simulink model "lab6"  (R2019a)
settings: Solver=VariableStepAuto  StartTime=0.0  StopTime=10.0  RelTol=1e-3
settings Model: Creator=sumli  LastModifiedBy=sumli

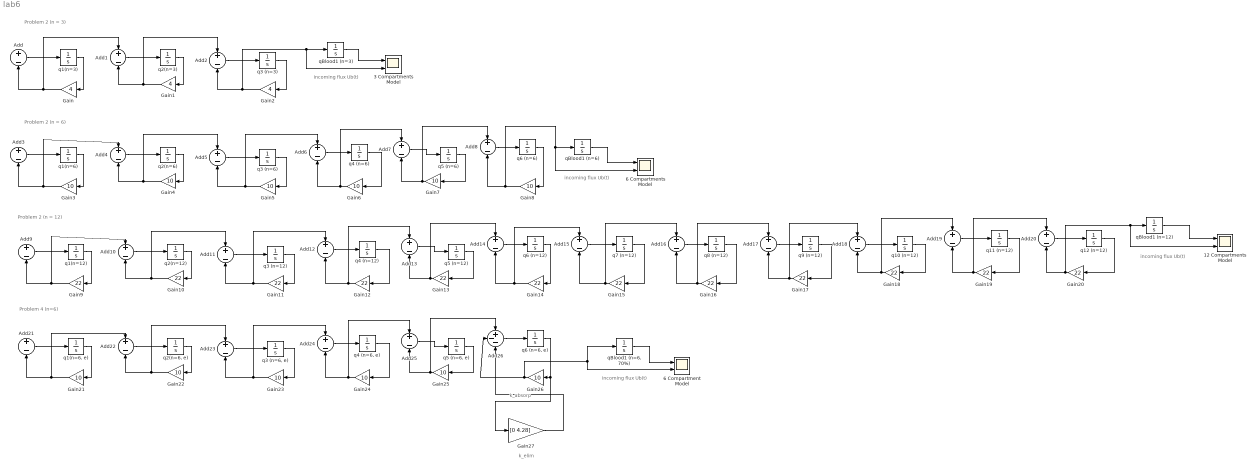
== system lab6 ==
  note: k_elim
  note: k_absorp
  note: incoming flux Ub(t)
  note: Problem 4 (n=6)
  note: Problem 2 (n = 12)
  note: Problem 2 (n = 6)
  note: Problem 2 (n = 3)
  note: incoming flux Ub(t)
  note: incoming flux Ub(t)
  note: incoming flux Ub(t)
  12 Compartments Model : Scope  NumInputPorts=2
  3 Compartments Model : Scope  NumInputPorts=2
  "6 Compartment Model " : Scope  NumInputPorts=2
  6 Compartments Model : Scope  NumInputPorts=2
  Add{,1..25} (26 alike) : Sum  Inputs=+-
  Add26 : Sum  Inputs=+--
  Gain : Gain  Gain=4
  Gain1 : Gain  Gain=4
  Gain{9..20} (12 alike) : Gain  Gain=22
  Gain2 : Gain  Gain=4
  Gain{3..8,21..26} (12 alike) : Gain  Gain=10
  Gain27 : Gain  Gain=[0 4.28]
  q1(n=12) : Integrator  InitialCondition=2
  q1(n=3) : Integrator  InitialCondition=2
  q1(n=6) : Integrator  InitialCondition=2
  "q1(n=6, e)" : Integrator  InitialCondition=2
  q10 (n=12) : Integrator
  q11 (n=12) : Integrator
  q12 (n=12) : Integrator
  q2(n=12) : Integrator
  q2(n=3) : Integrator
  q2(n=6) : Integrator
  "q2(n=6, e)" : Integrator
  q3 (n=12) : Integrator
  q3 (n=3) : Integrator
  q3 (n=6) : Integrator
  "q3 (n=6, e)" : Integrator
  q4 (n=12) : Integrator
  q4 (n=6) : Integrator
  "q4 (n=6, e)" : Integrator
  q5 (n=12) : Integrator
  q5 (n=6) : Integrator
  "q5 (n=6, e)" : Integrator
  q6 (n=12) : Integrator
  q6 (n=6) : Integrator
  "q6 (n=6, e)" : Integrator
  q7 (n=12) : Integrator
  q8 (n=12) : Integrator
  q9 (n=12) : Integrator
  qBlood1 (n=12) : Integrator
  qBlood1 (n=3) : Integrator
  qBlood1 (n=6) : Integrator
  "qBlood1 (n=6, 70%) " : Integrator
  wires:
  Add/1 -> q1(n=3)/1
  q1(n=3)/1 -> Gain/1
  Gain/1 -> Add1/1, Add/2
  Add1/1 -> q2(n=3)/1
  q2(n=3)/1 -> Gain1/1
  Gain1/1 -> Add2/1, Add1/2
  q3 (n=3)/1 -> Gain2/1
  Add2/1 -> q3 (n=3)/1
  Gain2/1 -> 3 Compartments Model/2, qBlood1 (n=3)/1, Add2/2
  qBlood1 (n=3)/1 -> 3 Compartments Model/1
  Gain3/1 -> Add4/1, Add3/2
  Add3/1 -> q1(n=6)/1
  Add5/1 -> q3 (n=6)/1
  Add4/1 -> q2(n=6)/1
  q3 (n=6)/1 -> Gain5/1
  q1(n=6)/1 -> Gain3/1
  q2(n=6)/1 -> Gain4/1
  Gain4/1 -> Add5/1, Add4/2
  Gain5/1 -> Add6/1, Add5/2
  qBlood1 (n=6)/1 -> 6 Compartments Model/1
  Add6/1 -> q4 (n=6)/1
  q4 (n=6)/1 -> Gain6/1
  Gain6/1 -> Add7/1, Add6/2
  Add7/1 -> q5 (n=6)/1
  q5 (n=6)/1 -> Gain7/1
  Gain7/1 -> Add8/1, Add7/2
  Add8/1 -> q6 (n=6)/1
  q6 (n=6)/1 -> Gain8/1
  Gain8/1 -> qBlood1 (n=6)/1, 6 Compartments Model/2, Add8/2
  q4 (n=12)/1 -> Gain12/1
  Add13/1 -> q5 (n=12)/1
  q3 (n=12)/1 -> Gain11/1
  Gain13/1 -> Add14/1, Add13/2
  Gain10/1 -> Add11/1, Add10/2
  Add12/1 -> q4 (n=12)/1
  q5 (n=12)/1 -> Gain13/1
  Add10/1 -> q2(n=12)/1
  Gain11/1 -> Add12/1, Add11/2
  q2(n=12)/1 -> Gain10/1
  Add11/1 -> q3 (n=12)/1
  Add9/1 -> q1(n=12)/1
  Add14/1 -> q6 (n=12)/1
  Gain9/1 -> Add10/1, Add9/2
  q1(n=12)/1 -> Gain9/1
  Gain14/1 -> Add15/1, Add14/2
  Gain12/1 -> Add13/1, Add12/2
  q6 (n=12)/1 -> Gain14/1
  Add15/1 -> q7 (n=12)/1
  q7 (n=12)/1 -> Gain15/1
  Gain15/1 -> Add16/1, Add15/2
  Add16/1 -> q8 (n=12)/1
  q8 (n=12)/1 -> Gain16/1
  Gain16/1 -> Add17/1, Add16/2
  Add17/1 -> q9 (n=12)/1
  q9 (n=12)/1 -> Gain17/1
  Gain17/1 -> Add18/1, Add17/2
  Add18/1 -> q10 (n=12)/1
  q10 (n=12)/1 -> Gain18/1
  Gain18/1 -> Add19/1, Add18/2
  Add19/1 -> q11 (n=12)/1
  q11 (n=12)/1 -> Gain19/1
  Gain19/1 -> Add20/1, Add19/2
  Add20/1 -> q12 (n=12)/1
  q12 (n=12)/1 -> Gain20/1
  Gain20/1 -> 12 Compartments Model/2, qBlood1 (n=12)/1, Add20/2
  qBlood1 (n=12)/1 -> 12 Compartments Model/1
  "q4 (n=6, e)"/1 -> Gain24/1
  Add25/1 -> "q5 (n=6, e)"/1
  "q3 (n=6, e)"/1 -> Gain23/1
  Gain25/1 -> Add26/1, Add25/2
  "qBlood1 (n=6, 70%) "/1 -> "6 Compartment Model "/1
  Gain22/1 -> Add23/1, Add22/2
  Add24/1 -> "q4 (n=6, e)"/1
  "q5 (n=6, e)"/1 -> Gain25/1
  Add22/1 -> "q2(n=6, e)"/1
  Gain23/1 -> Add24/1, Add23/2
  "q2(n=6, e)"/1 -> Gain22/1
  Add23/1 -> "q3 (n=6, e)"/1
  Add21/1 -> "q1(n=6, e)"/1
  Add26/1 -> "q6 (n=6, e)"/1
  Gain21/1 -> Add22/1, Add21/2
  "q1(n=6, e)"/1 -> Gain21/1
  Gain26/1 -> "qBlood1 (n=6, 70%) "/1, "6 Compartment Model "/2, Add26/2
  Gain24/1 -> Add25/1, Add24/2
  "q6 (n=6, e)"/1 -> Gain27/1, Gain26/1
  Gain27/1 -> Add26/3
